simulink model "gen_attitude_ref"  (R2019a)
settings: Solver=FixedStepAuto  StartTime=0.0  StopTime=100  FixedStep=0.01  RelTol=1e-3
settings Model: Creator=Duong  LastModifiedBy=Duong

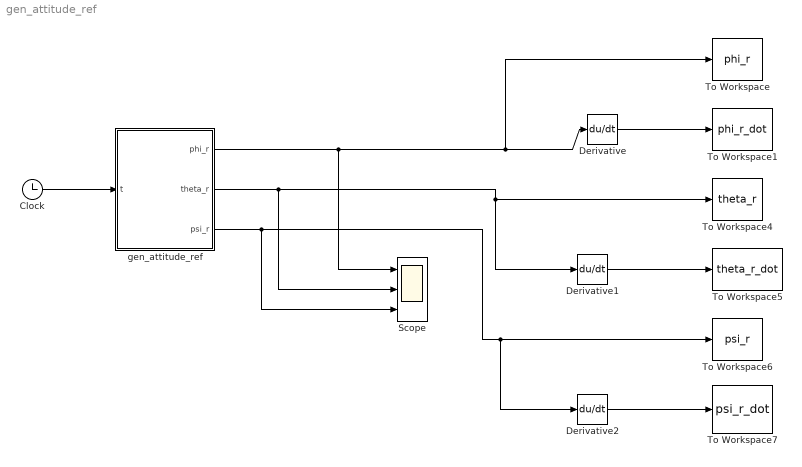
== system gen_attitude_ref ==
  Clock : Clock
  Derivative : Derivative
  Derivative1 : Derivative
  Derivative2 : Derivative
  Scope : Scope  NumInputPorts=3
  To Workspace : ToWorkspace  VariableName=phi_r  SampleTime=-1
      settings: Save2DSignal=2-D array (concatenate along first dimension)
  To Workspace1 : ToWorkspace  VariableName=phi_r_dot  SampleTime=-1
      settings: Save2DSignal=2-D array (concatenate along first dimension)
  To Workspace4 : ToWorkspace  VariableName=theta_r  SampleTime=-1
      settings: Save2DSignal=2-D array (concatenate along first dimension)
  To Workspace5 : ToWorkspace  VariableName=theta_r_dot  SampleTime=-1
      settings: Save2DSignal=2-D array (concatenate along first dimension)
  To Workspace6 : ToWorkspace  VariableName=psi_r  SampleTime=-1
      settings: Save2DSignal=2-D array (concatenate along first dimension)
  To Workspace7 : ToWorkspace  VariableName=psi_r_dot  SampleTime=-1
      settings: Save2DSignal=2-D array (concatenate along first dimension)
  gen_attitude_ref : MATLAB Function  TreatAsAtomicUnit=on
  wires:
  Clock/1 -> gen_attitude_ref/1(t)
  gen_attitude_ref/1(phi_r) -> Scope/1, To Workspace/1, Derivative/1
  Derivative/1 -> To Workspace1/1
  gen_attitude_ref/2(theta_r) -> Scope/2, To Workspace4/1, Derivative1/1
  Derivative1/1 -> To Workspace5/1
  gen_attitude_ref/3(psi_r) -> Scope/3, Derivative2/1, To Workspace6/1
  Derivative2/1 -> To Workspace7/1

== matlab function gen_attitude_ref/gen_attitude_ref ==
  data: t input; phi_r output; theta_r output; psi_r output
function [phi_r, theta_r, psi_r] = fcn(t)
a=0.8;
f=0.1;
phi_r=a*sin(2*pi*f*t)*exp(-0.8*t);
theta_r=a*sin(2*pi*f*t+pi/2)*exp(-0.8*t);
psi_r=a*sin(2*pi*f*t+1);
% phi_r=a*sin(2*pi*f*t);
% theta_r=a*cos(2*pi*f*t);
% psi_r=a*cos(2*pi*f*t+1);

psi_r=0;
